simulink model "new_nncACCsystem_5_50"  (R2021a)
(part 4 of 14)

  "IW{2,1}(50,:)'" : Constant  Value=[0.5876054829030852300064680093782953917980194091796875;-0.9360541339866459420449018580256961286067962646484375;0.051217120952734986050192134143799194134771823883056640625;0.74488624473523590285850559666869230568408966064453125;0.64249146745524488011369612650014460086822509765625;0.467219163483837796047026813539559952914714813232421875;0.7791587121598759768659192559425719082355499267578125;-0.80066295443368229456382323405705392360687255859375;-0.91710354159817075725413815234787762165069580078125;-0.07631475218328974408077414182116626761853694915771484375;0.9853642730546205985575625163619406521320343017578125;0.26403143013761809498873844859190285205841064453125;-0.7118426507375914535913352665374986827373504638671875;0.5972832020400689057026966111152432858943939208984375;-0.388300550134478950070615610457025468349456787109375;-0.448888725093049500980413313300232402980327606201171875;0.9822458624617314004723311882116831839084625244140625;-0.1687334495410990342634249827824532985687255859375;-0.0469104031879667981996817616163752973079681396484375;0.93402267132190797127577752689830958843231201171875;0.0633730912504857080147502301770146004855632781982421875;0.0035015037886749755813298179418779909610748291015625;0.0989546506821141758081239458988420665264129638671875;-0.2260547507601468331106531195473507978022098541259765625;-0.66040639688816760166645281060482375323772430419921875;-0.452197054557106958849743705286527983844280242919921875;0.10675854477820249932573659634726936928927898406982421875;-0.1550200408480575386960254036239348351955413818359375;0.79638007281385159163988873842754401266574859619140625;0.15870568837686571672662694254540838301181793212890625;0.5962615854118904490377417459967546164989471435546875;-0.3090347604456586960708364131278358399868011474609375;0.826093173892381127387807282502762973308563232421875;-0.090333833776380600966149359010159969329833984375;-0.9012071961402357000991969471215270459651947021484375;0.854963223443573117066307531786151230335235595703125;0.155591738915859811864805806180811487138271331787109375;-0.7867938087330801355534504182287491858005523681640625;0.0784604175829799188601754167393664829432964324951171875;0.82048687085877058944305417753639630973339080810546875;-0.55885939241167414959221559911384247243404388427734375;-0.5038516455960493356514007246005348861217498779296875;0.1677769646785136625766199358622543513774871826171875;0.2340184348834665473138016977827646769583225250244140625;-0.275210526991715109801361904828809201717376708984375;0.2216751031212114420032577299934928305447101593017578125;0.52530293793324833728775047347880899906158447265625;0.71417485337766828390471118837012909352779388427734375;0.49692607675155986424186949079739861190319061279296875;0.1115498530945513711021277458712575025856494903564453125]
      mask Display: e = 0.06;c1 = [120 150 230]/255;c2 = ([120 150 230]+0)/383;c3 = ([120 150 230]+128)/383;patch([0 1 1 0],[0 0 1 1],c1);patch([0 1 1 1-e 1-e 0+e],[0 0 1 1-e 0+e 0+e],c2);patch([0 0 1 1-e 0+e 0+e],[0 1 1 1-e 1-e 0+e],c3);plot([0 1 1 0 0],[0 0 1 1 0]);disp('weights');
  "IW{2,1}(6,:)'" : Constant  Value=[0.201381052004877769689983324497006833553314208984375;0.485850086443432527261165887466631829738616943359375;-0.4687585608429480910075426436378620564937591552734375;-0.260040751668246361560932200518436729907989501953125;0.412329768300442989215071065700612962245941162109375;0.2101231191212902249532135101617313921451568603515625;0.1294718374968766294585975629161112010478973388671875;-0.800651891556668271476837617228738963603973388671875;-0.08504441971741538708329244400374591350555419921875;0.5033397684436933250395895811379887163639068603515625;-0.3109053053727823812124597679940052330493927001953125;-0.41636619352186965414830410736612975597381591796875;0.9954765818265356447369640591205097734928131103515625;0.315788250765848044210315492819063365459442138671875;-0.7592682360838181043760641841799952089786529541015625;-0.853812041259362164424828733899630606174468994140625;0.713540250877187975930837637861259281635284423828125;-0.2720798976407239333497045663534663617610931396484375;0.37742483283320904519086980144493281841278076171875;-0.7240169125454445353540222640731371939182281494140625;0.7011517305173355918412880782852880656719207763671875;-0.058075301629038289519257887150160968303680419921875;-0.5794103235690115649703102462808601558208465576171875;-0.7766540202638221312980704169603995978832244873046875;0.5039593456550466310517322199302725493907928466796875;-0.588327640778256277798163864645175635814666748046875;-0.849799653388705333867392255342565476894378662109375;-0.319208710666914807774219298153184354305267333984375;0.13320608103908426755879190750420093536376953125;-0.9017520933989111586726039604400284588336944580078125;-0.825020600474092535847603357979096472263336181640625;-0.649317406892233606185982353053987026214599609375;0.04378306284339839038466379861347377300262451171875;-0.4746044421647155342469659444759599864482879638671875;0.300662534498110201042209155275486409664154052734375;0.9673582145273165178167573685641400516033172607421875;0.02000596281904076789714963524602353572845458984375;0.431867632986779437231916745076887309551239013671875;-0.4040669740847813162787360852234996855258941650390625;0.789149116737713374192253468208946287631988525390625;-0.042210597852486930747772930772043764591217041015625;0.615045665393918028485131799243390560150146484375;0.60283148138457942621926122228614985942840576171875;-0.271412477993162593037368424120359122753143310546875;-0.8241595121145375291149548502289690077304840087890625;-0.9561187926811400839000043561100028455257415771484375;-0.173694086495785438017946944455616176128387451171875;0.8254208072972810672496279948973096907138824462890625;-0.5230579817639104955873108337982557713985443115234375;-0.7685308122645027051333954659639857709407806396484375]
      mask Display: e = 0.06;c1 = [120 150 230]/255;c2 = ([120 150 230]+0)/383;c3 = ([120 150 230]+128)/383;patch([0 1 1 0],[0 0 1 1],c1);patch([0 1 1 1-e 1-e 0+e],[0 0 1 1-e 0+e 0+e],c2);patch([0 0 1 1-e 0+e 0+e],[0 1 1 1-e 1-e 0+e],c3);plot([0 1 1 0 0],[0 0 1 1 0]);disp('weights');
  "IW{2,1}(7,:)'" : Constant  Value=[0.4928698913827764815920318142161704599857330322265625;-0.76896079728071031755831654663779772818088531494140625;-0.71358251068255873494905472398386336863040924072265625;-0.65241481611493468140139384559006430208683013916015625;0.2300237087786433931579921363663743250072002410888671875;-0.81878763853863822941292482937569729983806610107421875;0.45451557614613957714055914038908667862415313720703125;-0.2921851389879004390337513541453517973423004150390625;0.7971660143829344402632841593003831803798675537109375;0.9758006675062722568014805801794864237308502197265625;0.06602807768526801346364862865812028758227825164794921875;0.2499638643127510828634285644511692225933074951171875;-0.4837148634458283691373026158544234931468963623046875;0.012960259352839502422494177835687878541648387908935546875;-0.4024255878880487191651127432123757898807525634765625;-0.249536894350515570106807672345894388854503631591796875;-0.802855394275903133660676758154295384883880615234375;0.7192777996515606897531824870384298264980316162109375;-0.083460992884685669679356578853912651538848876953125;-0.6962926648461589262950610645930282771587371826171875;-0.57438662235407489387029045246890746057033538818359375;0.6615860230893069182656063276226632297039031982421875;-0.97502630297658043900810298509895801544189453125;0.7750031335099947238376216773758642375469207763671875;0.99266250066038785870858873749966733157634735107421875;-0.07900260401891810724261944187674089334905147552490234375;-0.87029871190269136871364707985776476562023162841796875;0.833089510879824413080996237113140523433685302734375;-0.2622722844110516593474358160165138542652130126953125;0.7866432532659330956192889061640016734600067138671875;0.620495265555522035327840058016590774059295654296875;0.262027039548903051269235220388509333133697509765625;0.68092069397115384532526149996556341648101806640625;0.30267012864473752387084459769539535045623779296875;-0.56261594130692460513643027297803200781345367431640625;-0.401077555075733727107945014722645282745361328125;-0.278753895084464409226399084218428470194339752197265625;-0.08618558166804479725442433846183121204376220703125;-0.1788473148627990616521543643102631904184818267822265625;-0.375004769859344888605079404442221857607364654541015625;-0.614869830693172136903967839316464960575103759765625;-0.48136824667140720723779168110922910273075103759765625;-0.4984179658240417420955736815812997519969940185546875;-0.493095440464099254995744558982551097869873046875;0.432058053944118281020081440146896056830883026123046875;0.5301047311132014439039039643830619752407073974609375;-0.76235820885706129246273121680133044719696044921875;-0.725186176623851874722959109931252896785736083984375;0.76779272224313455108557491257670335471630096435546875;-0.347249748141330361050904684816487133502960205078125]
      mask Display: e = 0.06;c1 = [120 150 230]/255;c2 = ([120 150 230]+0)/383;c3 = ([120 150 230]+128)/383;patch([0 1 1 0],[0 0 1 1],c1);patch([0 1 1 1-e 1-e 0+e],[0 0 1 1-e 0+e 0+e],c2);patch([0 0 1 1-e 0+e 0+e],[0 1 1 1-e 1-e 0+e],c3);plot([0 1 1 0 0],[0 0 1 1 0]);disp('weights');
  "IW{2,1}(8,:)'" : Constant  Value=[0.516583426325593730865648467442952096462249755859375;0.5164855642357555343124886348959989845752716064453125;0.4988196040123653585141028088401071727275848388671875;-0.06116147217169594363372908674136851914227008819580078125;-0.638525883881182920731589547358453273773193359375;-0.38431123269811540144047512512770481407642364501953125;-0.048138363528707601990408448955349740572273731231689453125;0.8259553953685101479464947260566987097263336181640625;-0.358516716693216885847306230061803944408893585205078125;-0.160727405942299839125553262419998645782470703125;0.7562336508836526860477533773519098758697509765625;0.4404159594748637829297877033241093158721923828125;-0.718650262026375941104561206884682178497314453125;0.01317354900762239544587117734408820979297161102294921875;-0.2619954906637034230953986480017192661762237548828125;0.154366763450219490749759643222205340862274169921875;-0.62346963026538571028822843800298869609832763671875;0.0904918842215274299434213389758951961994171142578125;-0.4996593959594874956309240587870590388774871826171875;0.244392501153549712711310348822735249996185302734375;-0.385756546958892609922031624591909348964691162109375;-0.3803029328221836369294805990648455917835235595703125;0.245464475232142209648600328364409506320953369140625;0.31627883041677662401269799374858848750591278076171875;-0.220783112719417029534696439441177062690258026123046875;-0.4892060131587339100178724038414657115936279296875;0.297660946859123642926903130501159466803073883056640625;-0.786636705833117400032961086253635585308074951171875;-0.95078252278496133698126868694089353084564208984375;0.335014700769575402006239528418518602848052978515625;0.2360720462223564464210312507930211722850799560546875;-0.3088224140352548996446557794115506112575531005859375;0.4531284087184481723653561857645399868488311767578125;-0.7959513462381997417338652667240239679813385009765625;-0.9169591467970044096347237427835352718830108642578125;-0.0417567131602911700838376418687403202056884765625;-0.6077372800899514260208889027126133441925048828125;0.1234536867499034240580613186466507613658905029296875;0.136721423917505024991925210997578687965869903564453125;-0.933380201023525035708416908164508640766143798828125;0.9850378799329828627406868690741248428821563720703125;0.90323187457353604212784148330683819949626922607421875;0.1364322434356750601835983616183511912822723388671875;0.1602024987865380278861948681878857314586639404296875;0.2068341338276591390155090266489423811435699462890625;0.472882257836011898888273208285681903362274169921875;0.71120910985100493917343555949628353118896484375;-0.1320543164016661774606831158962449990212917327880859375;0.00634810122005052650251410994997058878652751445770263671875;0.5264539096202736079277428871137090027332305908203125]
      mask Display: e = 0.06;c1 = [120 150 230]/255;c2 = ([120 150 230]+0)/383;c3 = ([120 150 230]+128)/383;patch([0 1 1 0],[0 0 1 1],c1);patch([0 1 1 1-e 1-e 0+e],[0 0 1 1-e 0+e 0+e],c2);patch([0 0 1 1-e 0+e 0+e],[0 1 1 1-e 1-e 0+e],c3);plot([0 1 1 0 0],[0 0 1 1 0]);disp('weights');
  "IW{2,1}(9,:)'" : Constant  Value=[0.7311534984482737087319037527777254581451416015625;-0.56492040241266128219876918592490255832672119140625;0.478626862990769286199110865709371864795684814453125;0.15127334535331760090315356137580238282680511474609375;0.92159532562647428211022315736045129597187042236328125;-0.95525776024599451385910242606769315898418426513671875;-0.47532319767005926092195977616938762366771697998046875;0.7824933170535366411257882646168582141399383544921875;-0.92846766618789100533604141674004495143890380859375;0.5291007901973474591983404025086201727390289306640625;0.01213711489784217480158989843630479299463331699371337890625;-0.51388898085603873511217898339964449405670166015625;0.89087552171300388170749329219688661396503448486328125;-0.458980542747500386280279371931101195514202117919921875;-0.8493593767858438337015059005352668464183807373046875;0.1686748432012899756582413601790904067456722259521484375;0.7296327601544410068612478426075540482997894287109375;0.525915418169948356563736524549312889575958251953125;-0.9491644273004113951941462801187299191951751708984375;0.040314636789632936342275826291370321996510028839111328125;-0.2229909122890270378736232714800280518829822540283203125;-0.29382954320168952477843049564398825168609619140625;-0.725042243392566287951694903313182294368743896484375;0.496018664895358230015887102126725949347019195556640625;0.2191441043237924712894226786374929361045360565185546875;-0.87070780163357641701082911822595633566379547119140625;-0.412719949477278802429935922191361896693706512451171875;-0.7696505678752714185719696615706197917461395263671875;0.26437652548641843441856735807959921658039093017578125;-0.68360162857758932641871751911821775138378143310546875;-0.1837017675100780511598941302509047091007232666015625;-0.0403037933152223804000868767616339027881622314453125;0.8128257066634227978596527464105747640132904052734375;-0.2989129312523053361161373686627484858036041259765625;-0.69414256704407295561765067759552039206027984619140625;0.8266451383512281037013735840446315705776214599609375;0.8657246970052827617081447897362522780895233154296875;0.009305657392548294382095264154486358165740966796875;0.03750843369035931906818603920328314416110515594482421875;-0.3377539730839058673694808021537028253078460693359375;-0.9984682892684730859400588087737560272216796875;-0.59828975880366019879375016898848116397857666015625;0.869569033369367527797066941275261342525482177734375;0.446354729371927494430138949610409326851367950439453125;-0.858776275625421359194433534867130219936370849609375;0.2448992723879843680379053694196045398712158203125;0.1880218603817260802912869621650315821170806884765625;0.3977736947451326887659206477110274136066436767578125;0.6086580792140521278810183503082953393459320068359375;0.68805074319521997150417291777557693421840667724609375]
      mask Display: e = 0.06;c1 = [120 150 230]/255;c2 = ([120 150 230]+0)/383;c3 = ([120 150 230]+128)/383;patch([0 1 1 0],[0 0 1 1],c1);patch([0 1 1 1-e 1-e 0+e],[0 0 1 1-e 0+e 0+e],c2);patch([0 0 1 1-e 0+e 0+e],[0 1 1 1-e 1-e 0+e],c3);plot([0 1 1 0 0],[0 0 1 1 0]);disp('weights');
  Mux : Mux  Inputs=50
      mask Display: e = 0.06;c1 = [120 150 230]/255;c2 = ([120 150 230]+0)/383;c3 = ([120 150 230]+128)/383;patch([0 1 1 0],[0 0 1 1],c1);patch([0 1 1 1-e 1-e 0+e],[0 0 1 1-e 0+e 0+e],c2);patch([0 0 1 1-e 0+e 0+e],[0 1 1 1-e 1-e 0+e],c3);plot([0 1 1 0 0],[0 0 1 1 0]);disp('Mux');
  dotprod{1..50} (50 alike) : neural/Weight Functions/dotprod
  "lz{2,1}" : Outport
      mask Display: e = 0.06;c1 = [120 230 180]/255;c2 = ([120 230 180]+0)/(256+128);c3 = ([120 230 180]+128)/(256+128);patch([0 1 1 0],[0 0 1 1],c1);patch([0 1 1 1-e 1-e 0+e],[0 0 1 1-e 0+e 0+e],c2);patch([0 0 1 1-e 0+e 0+e],[0 1 1 1-e 1-e 0+e],c3);plot([0 1 1 0 0],[0 0 1 1 0]);
  wires:
  "IW{2,1}(1,:)'"/1 -> dotprod1/1
  "ad{2,1}"/1 -> dotprod1/2, dotprod2/2, dotprod3/2, dotprod4/2, dotprod5/2, dotprod6/2, dotprod7/2, dotprod8/2, dotprod9/2, dotprod10/2, dotprod11/2, dotprod12/2, dotprod13/2, dotprod14/2, dotprod15/2, dotprod16/2, dotprod17/2, dotprod18/2, dotprod19/2, dotprod20/2, dotprod21/2, dotprod22/2, dotprod23/2, dotprod24/2, dotprod25/2, dotprod26/2, dotprod27/2, dotprod28/2, dotprod29/2, dotprod30/2, dotprod31/2, dotprod32/2, dotprod33/2, dotprod34/2, dotprod35/2, dotprod36/2, dotprod37/2, dotprod38/2, dotprod39/2, dotprod40/2, dotprod41/2, dotprod42/2, dotprod43/2, dotprod44/2, dotprod45/2, dotprod46/2, dotprod47/2, dotprod48/2, dotprod49/2, dotprod50/2
  dotprod1/1 -> Mux/1
  "IW{2,1}(2,:)'"/1 -> dotprod2/1
  dotprod2/1 -> Mux/2
  "IW{2,1}(3,:)'"/1 -> dotprod3/1
  dotprod3/1 -> Mux/3
  "IW{2,1}(4,:)'"/1 -> dotprod4/1
  dotprod4/1 -> Mux/4
  "IW{2,1}(5,:)'"/1 -> dotprod5/1
  dotprod5/1 -> Mux/5
  "IW{2,1}(6,:)'"/1 -> dotprod6/1
  dotprod6/1 -> Mux/6
  "IW{2,1}(7,:)'"/1 -> dotprod7/1
  dotprod7/1 -> Mux/7
  "IW{2,1}(8,:)'"/1 -> dotprod8/1
  dotprod8/1 -> Mux/8
  "IW{2,1}(9,:)'"/1 -> dotprod9/1
  dotprod9/1 -> Mux/9
  "IW{2,1}(10,:)'"/1 -> dotprod10/1
  dotprod10/1 -> Mux/10
  "IW{2,1}(11,:)'"/1 -> dotprod11/1
  dotprod11/1 -> Mux/11
  "IW{2,1}(12,:)'"/1 -> dotprod12/1
  dotprod12/1 -> Mux/12
  "IW{2,1}(13,:)'"/1 -> dotprod13/1
  dotprod13/1 -> Mux/13
  "IW{2,1}(14,:)'"/1 -> dotprod14/1
  dotprod14/1 -> Mux/14
  "IW{2,1}(15,:)'"/1 -> dotprod15/1
  dotprod15/1 -> Mux/15
  "IW{2,1}(16,:)'"/1 -> dotprod16/1
  dotprod16/1 -> Mux/16
  "IW{2,1}(17,:)'"/1 -> dotprod17/1
  dotprod17/1 -> Mux/17
  "IW{2,1}(18,:)'"/1 -> dotprod18/1
  dotprod18/1 -> Mux/18
  "IW{2,1}(19,:)'"/1 -> dotprod19/1
  dotprod19/1 -> Mux/19
  "IW{2,1}(20,:)'"/1 -> dotprod20/1
  dotprod20/1 -> Mux/20
  "IW{2,1}(21,:)'"/1 -> dotprod21/1
  dotprod21/1 -> Mux/21
  "IW{2,1}(22,:)'"/1 -> dotprod22/1
  dotprod22/1 -> Mux/22
  "IW{2,1}(23,:)'"/1 -> dotprod23/1
  dotprod23/1 -> Mux/23
  "IW{2,1}(24,:)'"/1 -> dotprod24/1
  dotprod24/1 -> Mux/24
  "IW{2,1}(25,:)'"/1 -> dotprod25/1
  dotprod25/1 -> Mux/25
  "IW{2,1}(26,:)'"/1 -> dotprod26/1
  dotprod26/1 -> Mux/26
  "IW{2,1}(27,:)'"/1 -> dotprod27/1
  dotprod27/1 -> Mux/27
  "IW{2,1}(28,:)'"/1 -> dotprod28/1
  dotprod28/1 -> Mux/28
  "IW{2,1}(29,:)'"/1 -> dotprod29/1
  dotprod29/1 -> Mux/29
  "IW{2,1}(30,:)'"/1 -> dotprod30/1
  dotprod30/1 -> Mux/30
  "IW{2,1}(31,:)'"/1 -> dotprod31/1
  dotprod31/1 -> Mux/31
  "IW{2,1}(32,:)'"/1 -> dotprod32/1
  dotprod32/1 -> Mux/32
  "IW{2,1}(33,:)'"/1 -> dotprod33/1
  dotprod33/1 -> Mux/33
  "IW{2,1}(34,:)'"/1 -> dotprod34/1
  dotprod34/1 -> Mux/34
  "IW{2,1}(35,:)'"/1 -> dotprod35/1
  dotprod35/1 -> Mux/35
  "IW{2,1}(36,:)'"/1 -> dotprod36/1
  dotprod36/1 -> Mux/36
  "IW{2,1}(37,:)'"/1 -> dotprod37/1
  dotprod37/1 -> Mux/37
  "IW{2,1}(38,:)'"/1 -> dotprod38/1
  dotprod38/1 -> Mux/38
  "IW{2,1}(39,:)'"/1 -> dotprod39/1
  dotprod39/1 -> Mux/39
  "IW{2,1}(40,:)'"/1 -> dotprod40/1
  dotprod40/1 -> Mux/40
  "IW{2,1}(41,:)'"/1 -> dotprod41/1
  dotprod41/1 -> Mux/41
  "IW{2,1}(42,:)'"/1 -> dotprod42/1
  dotprod42/1 -> Mux/42
  "IW{2,1}(43,:)'"/1 -> dotprod43/1
  dotprod43/1 -> Mux/43
  "IW{2,1}(44,:)'"/1 -> dotprod44/1
  dotprod44/1 -> Mux/44
  "IW{2,1}(45,:)'"/1 -> dotprod45/1
  dotprod45/1 -> Mux/45
  "IW{2,1}(46,:)'"/1 -> dotprod46/1
  dotprod46/1 -> Mux/46
  "IW{2,1}(47,:)'"/1 -> dotprod47/1
  dotprod47/1 -> Mux/47
  "IW{2,1}(48,:)'"/1 -> dotprod48/1
  dotprod48/1 -> Mux/48
  "IW{2,1}(49,:)'"/1 -> dotprod49/1
  dotprod49/1 -> Mux/49
  "IW{2,1}(50,:)'"/1 -> dotprod50/1
  dotprod50/1 -> Mux/50
  Mux/1 -> "lz{2,1}"/1
